simulink model "base_closed_loop_model_PID_compare"  (R2017a)
settings: Solver=ode45  StartTime=0.0  StopTime=1  RelTol=1e-3  EnableMultiTasking=on
settings Model: Creator=cpmcclel  LastModifiedBy=cpmcclel
settings DataIOCC: LimitDataPoints=on  SaveFormat=Array
settings OptimizationCC: LifeSpan=inf
settings DebuggingCC: SolverPrmCheckMsg=warning  SFUnexpectedBacktrackingDiag=warning  SFNoUnconditionalDefaultTransitionDiag=warning  SFExecutionAtInitializationDiag=none
settings HardwareCC: ProdBitPerPointer=32  ProdBitPerSizeT=32  ProdBitPerPtrDiffT=32  ProdLargestAtomicFloat=None  ProdIntDivRoundTo=Undefined  ProdEndianess=Unspecified  ProdWordSize=32  ProdHWDeviceType=32-bit Generic
settings ModelReferenceCC: PropagateSignalLabelsOutOfModel=off
settings GRTTargetCC: TargetLangStandard=C89/C90 (ANSI)  GeneratePreprocessorConditionals=Disable all
settings ConfigComp: CovMetricSettings=dw  CovHtmlReporting=on  CovSaveCumulativeToWorkspaceVar=on  CovSaveSingleToWorkspaceVar=on  CovExternalEMLEnable=off  CovSFcnEnable=off

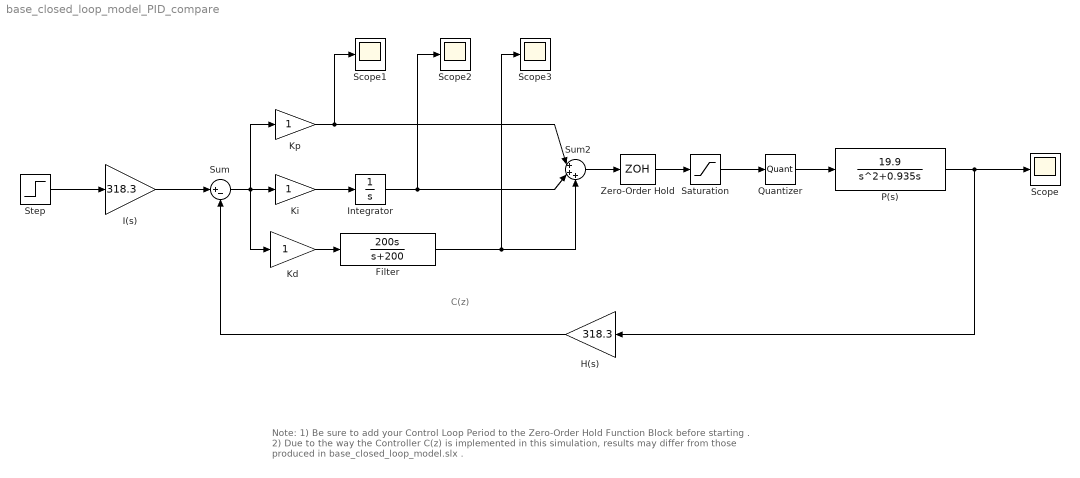
== system base_closed_loop_model_PID_compare ==
  note: Note:
      | 1) Be sure to add your Control Loop Period to the Zero-Order Hold Function Block before starting .
      | 2) Due to the way the Controller C(z) is implemented in this simulation, results may differ from
      | those produced in base_closed_loop_model.slx .
  note: C(z)
  Filter : TransferFcn  Numerator=[200 0 ]  Denominator=[1 200]
  H(s) : Gain  Gain=318.3
  I(s) : Gain  Gain=318.3
  Integrator : Integrator
  Kd : Gain
  Ki : Gain
  Kp : Gain
  P(s) : TransferFcn  Numerator=[19.9]  Denominator=[1 0.935 0]
  Quantizer : Quantizer  QuantizationInterval=12/1023
  Saturation : Saturate  UpperLimit=12  LowerLimit=-12
  Scope{,1..3} (4 alike) : Scope
  Step : Step  Time=0
  Sum : Sum  Inputs=|+-
  Sum2 : Sum  Inputs=|+++
  Zero-Order Hold : ZeroOrderHold  SampleTime=-1
  wires:
  Step/1 -> I(s)/1
  Kd/1 -> Filter/1
  Sum/1 -> Kd/1, Ki/1, Kp/1
  Ki/1 -> Integrator/1
  Integrator/1 -> Sum2/2, Scope2/1
  Kp/1 -> Sum2/1, Scope1/1
  Filter/1 -> Scope3/1, Sum2/3
  Sum2/1 -> Zero-Order Hold/1
  P(s)/1 -> H(s)/1, Scope/1
  Saturation/1 -> Quantizer/1
  H(s)/1 -> Sum/2
  I(s)/1 -> Sum/1
  Quantizer/1 -> P(s)/1
  Zero-Order Hold/1 -> Saturation/1
